simulink model "TD1_b"  (R2024b)
settings: Solver=VariableStepAuto  StartTime=0.0  StopTime=10.0  RelTol=1e-3
settings Model: Creator=simon  LastModifiedBy=simon

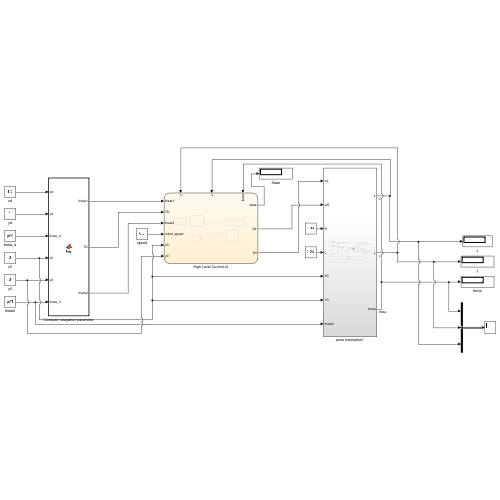
[thumbnail: Simulink's stored preview of the top-level diagram]
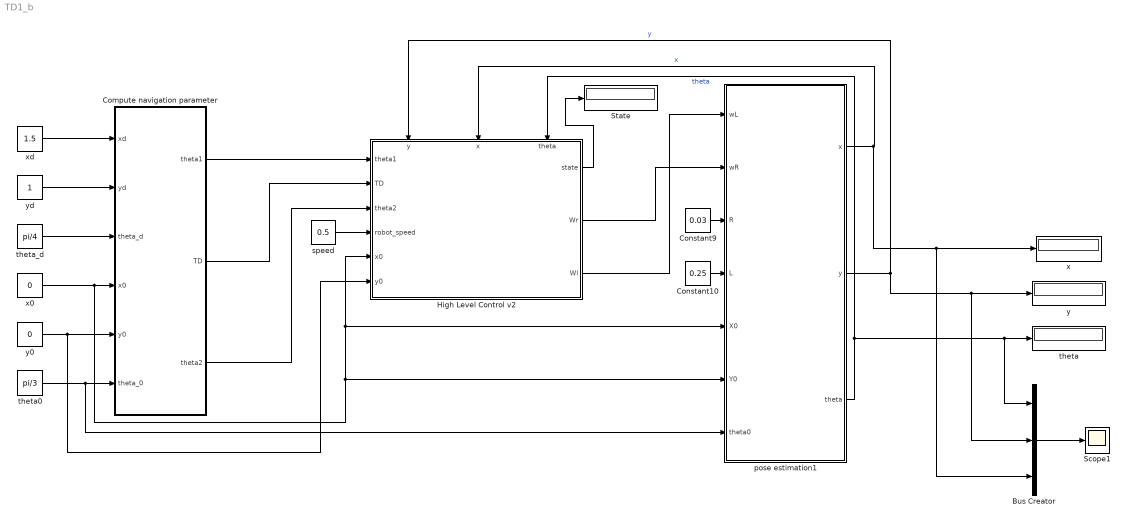
== system TD1_b ==
  Bus Creator : BusCreator  Inputs=3
  Compute navigation parameter : MATLAB Function  TreatAsAtomicUnit=on
  Constant10 : Constant  Value=0.25
  Constant9 : Constant  Value=0.03
  High Level Control v2 : Stateflow chart  TreatAsAtomicUnit=on
      settings: PortSchema="{\"entries\":[{\"content\":{\"sides\":[{\"content\":{\"connectorIds\":[\"In6\",\"In2\",\"In3\",\"In7\",\"In8\",\"In9\"]},\"type\":\"ConnectorPlacement.EquallySpacedRectSide\",\"uuid\":\"c86bd203-b0ab-41aa-b914-bef04ced142d\"},{\"content\":{\"connectorIds\":[\"Out1\",\"Out2\",\"Out3\"],\"side\":\"RIGHT\"},\"type\":\"ConnectorPlacement.EquallySpacedRectSide\",\"uuid\":\"adc4a676-1c74-4ba4-992a-015d2aed7172\"},{\"content\":{\"connectorIds\":[\"In1\",\"In4\",\"In5\"],\"side\":\"TOP\"},\"type\":\"ConnectorPlacement.EquallySpacedRectSide\",\"uuid\":\"7d3f68d4-35f9-4096-8fe1-768046eca6e9\"}]},\"type\":\"ConnectorPlacement.EquallySpacedConnector\",\"uuid\":\"bcc88c28-889d-4cca-af5e-634e70de4cbc\"}],\"packageUris\":[\"http://schema.mathworks.com/mf0/Connector/R2020b\"],\"version\":\"1.0\"}"
  Scope1 : Scope
  State : Display
  pose estimation1 : Subsystem
  speed : Constant  Value=0.5
  theta : Display
  theta0 : Constant  Value=pi/3
  theta_d : Constant  Value=pi/4
  x : Display
  x0 : Constant  Value=0
  xd : Constant  Value=1.5
  y : Display
  y0 : Constant  Value=0
  yd : Constant
  wires:
  Bus Creator/1 -> Scope1/1
  pose estimation1/2(y) -> High Level Control v2/1(y), Bus Creator/2, y/1  "y"
  Constant9/1 -> pose estimation1/3(R)
  High Level Control v2/2(Wr) -> pose estimation1/2(wR)
  speed/1 -> High Level Control v2/7(robot_speed)
  Constant10/1 -> pose estimation1/4(L)
  High Level Control v2/1(state) -> State/1
  pose estimation1/1(x) -> Bus Creator/3, x/1, High Level Control v2/4(x)  "x"
  Compute navigation parameter/3(theta2) -> High Level Control v2/3(theta2)
  xd/1 -> Compute navigation parameter/1(xd)
  y0/1 -> High Level Control v2/9(y0), Compute navigation parameter/5(y0)
  Compute navigation parameter/1(theta1) -> High Level Control v2/6(theta1)
  pose estimation1/3(theta) -> Bus Creator/1, theta/1, High Level Control v2/5(theta)  "theta"
  yd/1 -> Compute navigation parameter/2(yd)
  theta0/1 -> Compute navigation parameter/6(theta_0), pose estimation1/7(theta0)
  theta_d/1 -> Compute navigation parameter/3(theta_d)
  High Level Control v2/3(Wl) -> pose estimation1/1(wL)
  x0/1 -> pose estimation1/6(Y0), pose estimation1/5(X0), High Level Control v2/8(x0), Compute navigation parameter/4(x0)
  Compute navigation parameter/2(TD) -> High Level Control v2/2(TD)

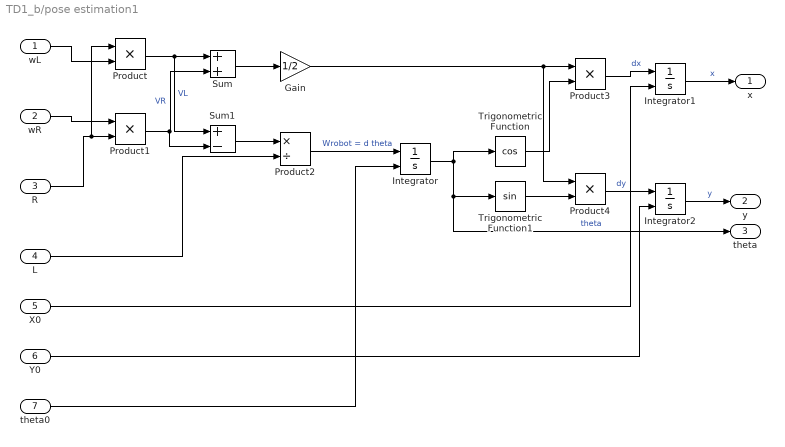
== system TD1_b/pose estimation1 ==
  wL : Inport
  wR : Inport  Port=2
  R : Inport  Port=3
  L : Inport  Port=4
  X0 : Inport  Port=5
  Y0 : Inport  Port=6
  theta0 : Inport  Port=7
  Gain : Gain  Gain=1/2
  Integrator : Integrator  InitialConditionSource=external
  Integrator1 : Integrator  InitialConditionSource=external
  Integrator2 : Integrator  InitialConditionSource=external
  Product{,1,3..4} (4 alike) : Product
  Product2 : Product  Inputs=*/
  Sum : Sum
  Sum1 : Sum  Inputs=+-
  Trigonometric Function : Trigonometry  Operator=cos
  Trigonometric Function1 : Trigonometry
  x : Outport
  y : Outport  Port=2
  theta : Outport  Port=3
  wires:
  L/1 -> Product2/2
  Integrator2/1 -> y/1  "y"
  Trigonometric Function/1 -> Product3/2
  Trigonometric Function1/1 -> Product4/2
  Gain/1 -> Product4/1, Product3/1
  Product3/1 -> Integrator1/1  "dx"
  R/1 -> Product/1, Product1/2
  Sum1/1 -> Product2/1
  Product2/1 -> Integrator/1  "Wrobot = d theta"
  Sum/1 -> Gain/1
  Product4/1 -> Integrator2/1  "dy"
  Integrator1/1 -> x/1  "x"
  Integrator/1 -> Trigonometric Function/1, Trigonometric Function1/1, theta/1  "theta"
  Product/1 -> Sum1/1, Sum/1  "VL"
  Product1/1 -> Sum1/2, Sum/2  "VR"
  wL/1 -> Product/2
  wR/1 -> Product1/1
  X0/1 -> Integrator1/2
  Y0/1 -> Integrator2/2
  theta0/1 -> Integrator/2

== matlab function TD1_b/Compute navigation parameter ==
  data: xd input; theta1 output; TD output; yd input; theta_d input; theta2 output; x0 input; y0 input; theta_0 input
function [theta1, TD, theta2] = fcn(xd, yd, theta_d, x0, y0, theta_0)

TD = sqrt((xd-x0).^2+ (yd-y0).^2);

theta1 = sign(yd - y0).*acos((xd-x0)/TD)-theta_0;
theta2 = theta_d - (theta1 + theta_0);

== stateflow chart TD1_b/High Level Control v2 ==
  state state1
    entry: state= 1;
    during:
    if (theta1 > 0)
    Wl = robot_speed;
    Wr = -robot_speed;
    else
    Wl = -robot_speed;
    Wr = robot_speed;
    end
  state state0
    entry:state= 0;
    theta_o = theta;
    angleObjectif = theta_o + theta1;
  state state2
    entry: state= 2;
    during:
    Wl = robot_speed;
    Wr = robot_speed;
  state state3
    entry: state= 3;
    during:
    if (theta2 < 0)
    Wl = robot_speed;
    Wr = -robot_speed;
    else
    Wl = -robot_speed;
    Wr = robot_speed;
    end
  state state4
    entry:
    Wl = 0;
    Wr = 0;
    state= 4;
  (default) -> state0
  state0 -> state1
  state1 -> state2 : [(theta1 > 0 && abs(theta- angleObjectif) <= 0.25) || (theta1 < 0 && abs(theta - angleObjectif) <= 0.25) ]
      | {Wl = 0; Wr = 0;}
  state2 -> state3 : [abs(sqrt((x-x0).^2 + (y-y0).^2) - TD) <= 0.1 || sqrt((x-x0).^2 + (y-y0).^2) > TD]
  state3 -> state4 : [abs(theta-theta2) <= 0.5]
  data: y input; TD input; theta2 input; x input; theta input; theta1 input; robot_speed input; state output; Wr output; Wl output; x0 input; y0 input; theta_o local double; angleObjectif local
